simulink model "Simulink_templates"  (R2025a)
settings: Solver=VariableStepAuto  StartTime=0.0  StopTime=10  FixedStep=pas  RelTol=1e-3
undefined symbols (not defined in the file): bool, controller, dt_realtime, pert
libraries: aerolibanimutils x2, cstblocks x1, simulink x1, sim3dlib x1, uavsim3dlib x1
settings Model: Creator=blaze8871  LastModifiedBy=adrien
settings SolverCC: AlgebraicLoopSolver=TrustRegion
settings DataIOCC: SignalLogging=off  DSMLogging=off
settings DebuggingCC: UnconnectedInputMsg=warning  UnconnectedOutputMsg=warning  UnconnectedLineMsg=warning
settings ModelReferenceCC: EnableRefExpFcnMdlSchedulingChecks=on
settings RTWCC: GPUComputeCapability=3.5

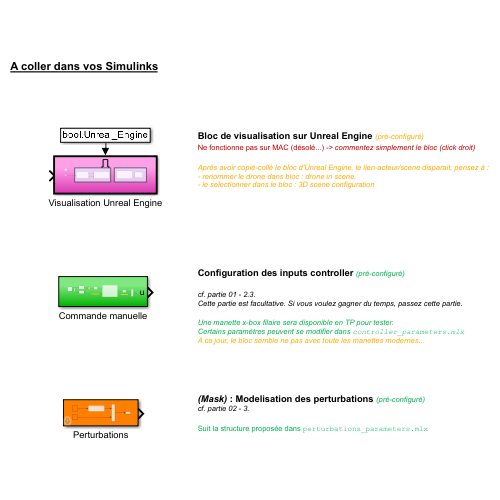
[thumbnail: Simulink's stored preview of the top-level diagram]
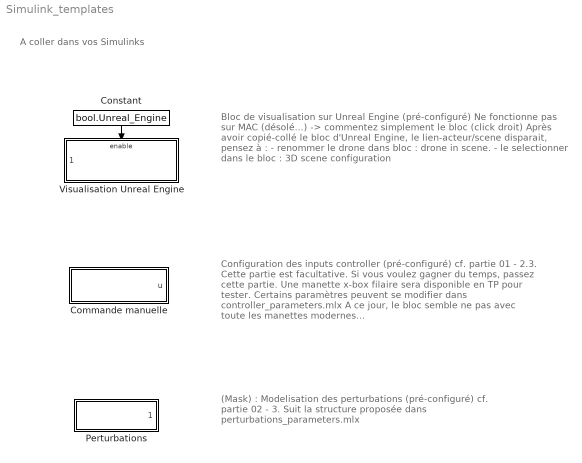
== system Simulink_templates ==
  note: A coller dans vos Simulinks
  note: Bloc de visualisation sur Unreal Engine (pré-configuré)
      | Ne fonctionne pas sur MAC (désolé...) -> commentez simplement le bloc (click droit)
      |
      | Après avoir copié-collé le bloc d'Unreal Engine, le lien-acteur/scene disparait, pensez à :
      | - renommer le drone dans bloc : drone in scene.
      | - le selectionner dans le bloc : 3D scene configuration
  note: Configuration des inputs controller (pré-configuré)
      |
      | cf. partie 01 - 2.3.
      | Cette partie est facultative. Si vous voulez gagner du temps, passez cette partie.
      |
      | Une manette x-box filaire sera disponible en TP pour tester.
      | Certains paramètres peuvent se modifier dans controller_parameters.mlx
      | A ce jour, le bloc semble ne pas avec toute les manettes modernes...
  note: (Mask) : Modelisation des perturbations (pré-configuré)
      | cf. partie 02 - 3.
      |
      | Suit la structure proposée dans perturbations_parameters.mlx
  Commande manuelle : Subsystem
  Constant : Constant  Value=bool.Unreal_Engine
  Perturbations : Subsystem  mask{perturbation=pert.motor, Ts=dt_realtime}
      mask prompts: perturbation "modèle de perturbation"; Ts "echantillonage"
      mask DialogControl ParameterGroupVar Prompt: Configuration - bruit blanc filtré
  Visualisation Unreal Engine : Subsystem
  wires:
  Constant/1 -> Visualisation Unreal Engine/Enable

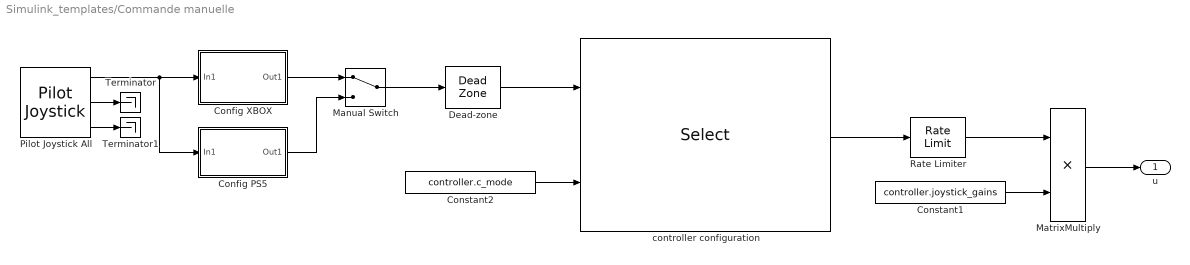
== system Simulink_templates/Commande manuelle ==
  Config PS5 : Subsystem
      mask Display: image('controller_ps5.png', [2,2,2,2,100,100]);
  "Config XBOX " : Subsystem
      mask Display: image('controller_xbox.png', [2,2,2,2,100,100]);
  Constant1 : Constant  Value=controller.joystick_gains
  Constant2 : Constant  Value=controller.c_mode
  Dead-zone : DeadZone  LowerValue=-0.2  UpperValue=0.2
  Manual Switch : ManualSwitch
  MatrixMultiply : Product
  Pilot Joystick All : aerolibanimutils/Pilot Joystick  JoystickID=Joystick1  OutputConfiguration=AllOutputs  SampleTime=dt_realtime
      settings: LibrarySourceBlock=aerolibanimutils/Pilot Joystick All
  "Rate Limiter " : RateLimiter  RisingSlewLimit=controller.rate_limits  FallingSlewLimit=-controller.rate_limits
  Terminator : Terminator
  Terminator1 : Terminator
  controller configuration : Selector  InputPortWidth=4  IndexOptions=Index vector (port)  Indices=[2 4 3 1]  OutputSizes=1
      mask Display: image('controller_modes.png');
  u : Outport
  wires:
  controller configuration/1 -> "Rate Limiter "/1
  MatrixMultiply/1 -> u/1
  Constant1/1 -> MatrixMultiply/2
  Constant2/1 -> controller configuration/2
  "Rate Limiter "/1 -> MatrixMultiply/1
  Dead-zone/1 -> controller configuration/1
  Pilot Joystick All/1 -> "Config XBOX "/1(In1), Config PS5/1(In1)
  Manual Switch/1 -> Dead-zone/1
  "Config XBOX "/1(Out1) -> Manual Switch/1
  Config PS5/1(Out1) -> Manual Switch/2
  Pilot Joystick All/2 -> Terminator/1
  Pilot Joystick All/3 -> Terminator1/1

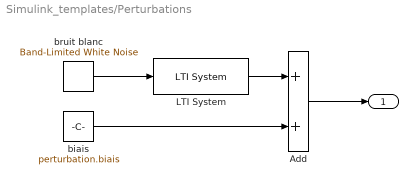
== system Simulink_templates/Perturbations ==
  Add : Sum
  LTI System : cstblocks/LTI System  sys=perturbation.filtre  IC=[]  PadeOrder=0
  biais : Constant  Value=perturbation.biais  SampleTime=Ts
  bruit blanc : simulink/Sources/Band-Limited White Noise  Cov=perturbation.noise_power  Ts=Ts  seed=perturbation.seed
  "  " : Outport
  wires:
  Add/1 -> "  "/1
  biais/1 -> Add/2
  LTI System/1 -> Add/1
  bruit blanc/1 -> LTI System/1

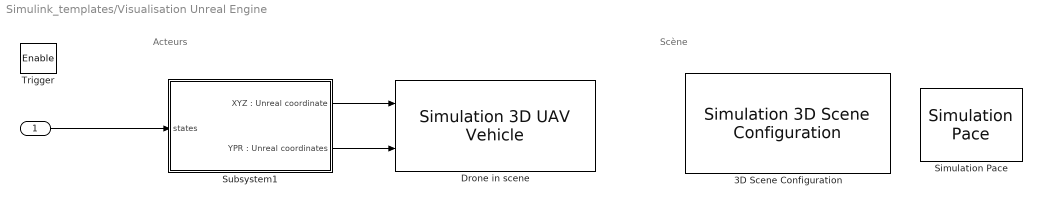
== system Simulink_templates/Visualisation Unreal Engine ==
  note: Acteurs
  note: Scène
  " " : Inport
  Trigger : EnablePort
  3D Scene Configuration : sim3dlib/Simulation 3D Scene Configuration  Priority=0  ProjectFormat=Default Scenes  SceneDesc=US city block  ProjectName=C:\Program Files\MATLAB\R2025a\toolbox\shared\sim3d_projects\automotive_project_windows\UE\WindowsNoEditor\VehicleSimulation.exe  ScenePath=/Game/Maps/USCityBlock  EnableOpenDRIVE=off  vehTagList={'Custom';'Scene Origin';'donnez_moi_un_nom'}  vehTag=donnez_moi_un_nom  AttachedCameraRelativeTranslation=[0 0 0]  FreeCameraDefaultInitialTranslation=[-6, 0, 2]  AttachedCameraRelativeRotation=[0 0 0]  FreeCameraDefaultInitialRotation=[0, -15, 0]  ViewpointName=Custom  FreeCameraInitialTranslation=[0 0 0]  ViewpointTranslation=[0 0 0]  FreeCameraInitialRotation=[0 0 0]  ViewpointRotation=[0 0 0]  OpVisEn=off  Ts=dt_realtime  EnableWindow=on  EnableRemoteAccess=off  EnableWeather=off  SunAzimuth=90  SunAltitude=40.0  EnableGeospatialSun=off  Latitude=0  Longitude=0  Date=2023-01-01  Time=10:30:00  GeoTimeZone=-5.0  SunDaylightSaving=off  wind=1  clouds=10  EnableVolumetricClouds=off  CloudCoverage=0  CloudAltitude=6  fog=0  rain=0  RaindropsEffect=off  SnowDensity=0  EnableGeospatial=off  TilesetSource=Earth terrain  UseTrueOrigin=off  OriginHeight=200  OriginLatitude=40.744652  OriginLongitude=-73.988864  MapStyle=Aerial  AdditionalAssetIDs=[]  UseAdvancedSunSky=off  SolarTime=11  TimeZone=-5  Day=21  Month=9  Year=2022  UseDaylightSavingTime=on  DSTStartDay=10  DSTStartMonth=3  DSTEndDay=3  DSTEndMonth=11  DSTSwitchHour=2  sensorTag=MainCamera1  sensorId=1  sensorName=MainCamera1  mountLoc=Origin  offsetFlag=off  tmountOffset=[0, 0, 0]  rmountOffset=[0, 0, 0]  HorizontalResolution=1280  VerticalResolution=720  HorizontalFOV=60  mountPoint=[0 0 0]  mountOrientation=[0 0 0]  aMode=4  ID=1  GeoTrigger=Inactive  ViewNameList={'Custom'}  ViewTranslationList={'[0 0 0]'}  ViewRotationList={'[0 0 0]'}
      settings: LibrarySourceBlock=uavsim3dlib/Simulation 3D Scene Configuration
  Drone in scene : uavsim3dlib/Simulation 3D UAV Vehicle  Priority=-1  Mesh=Quadrotor  MeshPath=/MathWorksUAVContent/UAVs/HexaRotorUAV/HexaRotor.HexaRotor  Color=Black  ActorName=donnez_moi_un_nom  UseGlobalFrame=off  InitialTranslation=[0 0 0]  InitialRotation=[0 0 0]  InitialTranslationGlobal=[0 0 0]  InitialGeoOrigin=[0 0 0]  InitialRotationGlobal=[0 0 0]  SampleTime=-1  ActorType=SimulinkVehicle  ID=C  aMode=4  ActorTag=donnez_moi_un_nom
  Simulation Pace : aerolibanimutils/Simulation Pace  SimulationPace=1  SleepMode=Auto  OutputPaceError=off  SampleTime=dt_realtime
  Subsystem1 : Subsystem
  wires:
  " "/1 -> Subsystem1/1(states)
  Subsystem1/1("XYZ : Unreal coordinate") -> Drone in scene/1
  Subsystem1/2("YPR : Unreal coordinates") -> Drone in scene/2

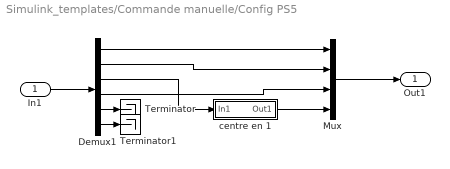
== system Simulink_templates/Commande manuelle/Config PS5 ==
  In1 : Inport
  Demux1 : Demux  Outputs=6
  Mux : Mux
  Terminator : Terminator
  Terminator1 : Terminator
  centre en 1 : Subsystem
  Out1 : Outport
  wires:
  Demux1/6 -> Terminator1/1
  Demux1/5 -> Terminator/1
  Demux1/4 -> Mux/3
  In1/1 -> Demux1/1
  Demux1/1 -> Mux/1
  Demux1/2 -> Mux/2
  Mux/1 -> Out1/1
  centre en 1/1(Out1) -> Mux/4
  Demux1/3 -> centre en 1/1(In1)

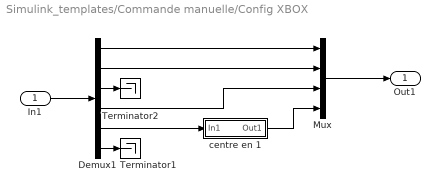
== system Simulink_templates/Commande manuelle/Config XBOX  ==
  In1 : Inport
  Demux1 : Demux  Outputs=6
  Mux : Mux
  Terminator1 : Terminator
  Terminator2 : Terminator
  centre en 1 : Subsystem
  Out1 : Outport
  wires:
  Mux/1 -> Out1/1
  Demux1/2 -> Mux/2
  Demux1/1 -> Mux/1
  In1/1 -> Demux1/1
  Demux1/6 -> Terminator1/1
  Demux1/4 -> Mux/3
  centre en 1/1(Out1) -> Mux/4
  Demux1/5 -> centre en 1/1(In1)
  Demux1/3 -> Terminator2/1

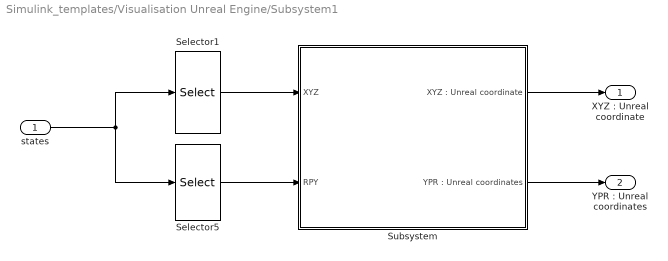
== system Simulink_templates/Visualisation Unreal Engine/Subsystem1 ==
  states : Inport
  Selector1 : Selector  InputPortWidth=12  IndexOptions=Index vector (dialog)  Indices=[1 3 5]  OutputSizes=1
  Selector5 : Selector  InputPortWidth=12  IndexOptions=Index vector (dialog)  Indices=[7 9 11]  OutputSizes=1
  Subsystem : Subsystem
  "XYZ : Unreal coordinate" : Outport
  "YPR : Unreal coordinates" : Outport  Port=2
  wires:
  states/1 -> Selector1/1, Selector5/1
  Subsystem/1("XYZ : Unreal coordinate") -> "XYZ : Unreal coordinate"/1
  Selector5/1 -> Subsystem/2(RPY)
  Subsystem/2("YPR : Unreal coordinates") -> "YPR : Unreal coordinates"/1
  Selector1/1 -> Subsystem/1(XYZ)

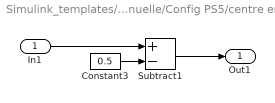
== system Simulink_templates/Commande manuelle/Config PS5/centre en 1 ==
  In1 : Inport
  Constant3 : Constant  Value=0.5
  Subtract1 : Sum  Inputs=+-
  Out1 : Outport
  wires:
  Subtract1/1 -> Out1/1
  In1/1 -> Subtract1/1
  Constant3/1 -> Subtract1/2

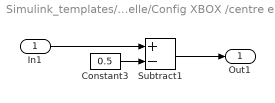
== system Simulink_templates/Commande manuelle/Config XBOX /centre en 1 ==
  In1 : Inport
  Constant3 : Constant  Value=0.5
  Subtract1 : Sum  Inputs=+-
  Out1 : Outport
  wires:
  Subtract1/1 -> Out1/1
  In1/1 -> Subtract1/1
  Constant3/1 -> Subtract1/2

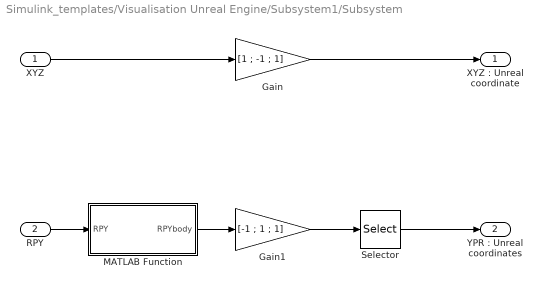
== system Simulink_templates/Visualisation Unreal Engine/Subsystem1/Subsystem ==
  XYZ : Inport
  RPY : Inport  Port=2
  Gain : Gain  Gain=[1 ; -1 ; 1]
  Gain1 : Gain  Gain=[-1 ; 1 ; 1]
  MATLAB Function : MATLAB Function  TreatAsAtomicUnit=on
  Selector : Selector  InputPortWidth=3  IndexOptions=Index vector (dialog)  Indices=[3 2 1]  OutputSizes=1
  "XYZ : Unreal coordinate" : Outport
  "YPR : Unreal coordinates" : Outport  Port=2
  wires:
  Gain1/1 -> Selector/1
  RPY/1 -> MATLAB Function/1(RPY)
  MATLAB Function/1(RPYbody) -> Gain1/1
  Selector/1 -> "YPR : Unreal coordinates"/1
  XYZ/1 -> Gain/1
  Gain/1 -> "XYZ : Unreal coordinate"/1

== matlab function Simulink_templates/Visualisation Unreal Engine/Subsystem1/Subsystem/MATLAB Function ==
  data: RPY input; RPYbody output
function RPYbody = fcn(RPY)


RX = [[1 0 0];...
       [0 cos(RPY(1)) -sin(RPY(1))];...
       [0 sin(RPY(1)) cos(RPY(1))]];

RY = [[cos(RPY(2)) 0 sin(RPY(2))];...
       [0 1 0];...
       [-sin(RPY(2)) 0 cos(RPY(2))]];

RZ = [[cos(RPY(3)) -sin(RPY(3)) 0];...
       [sin(RPY(3)) cos(RPY(3)) 0];...
       [0 0 1]];

RPYbody = inv(RZ*RY*RX)*RPY;
